simulink model "task2"  (R2023a)
settings: Solver=VariableStepAuto  StartTime=0.0  StopTime=10.0  RelTol=1e-3
settings Model: Creator=17634948724  LastModifiedBy=17634948724

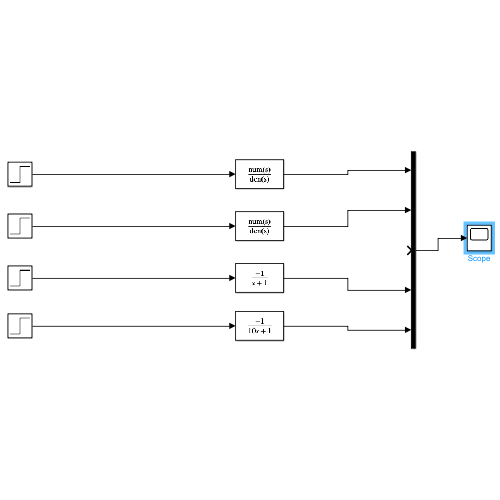
[thumbnail: Simulink's stored preview of the top-level diagram]
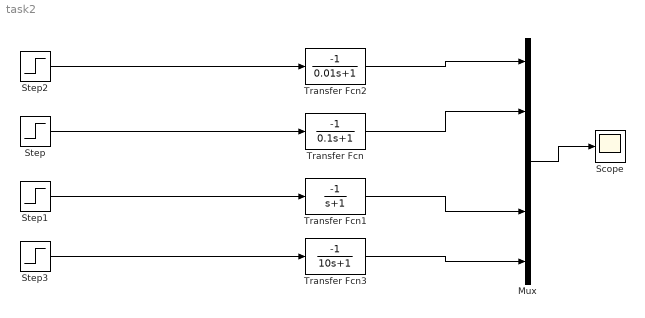
== system task2 ==
  Mux : Mux  Inputs=5
  Scope : Scope
  Step{,1..3} (4 alike) : Step  SampleTime=0
  Transfer Fcn : TransferFcn  Numerator=[-1]  Denominator=[0.1 1]
  Transfer Fcn1 : TransferFcn  Numerator=[-1]  Denominator=[1 1]
  Transfer Fcn2 : TransferFcn  Numerator=[-1]  Denominator=[0.01 1]
  Transfer Fcn3 : TransferFcn  Numerator=[-1]  Denominator=[10 1]
  wires:
  Step/1 -> Transfer Fcn/1
  Step1/1 -> Transfer Fcn1/1
  Step2/1 -> Transfer Fcn2/1
  Step3/1 -> Transfer Fcn3/1
  Mux/1 -> Scope/1
  Transfer Fcn2/1 -> Mux/1
  Transfer Fcn1/1 -> Mux/4
  Transfer Fcn/1 -> Mux/2
  Transfer Fcn3/1 -> Mux/5
